simulink model "pendulum_on_cart"  (R2022a)
settings: Solver=VariableStepAuto  StartTime=0.0  StopTime=20  RelTol=1e-3
settings Model: Creator=Home  LastModifiedBy=Home

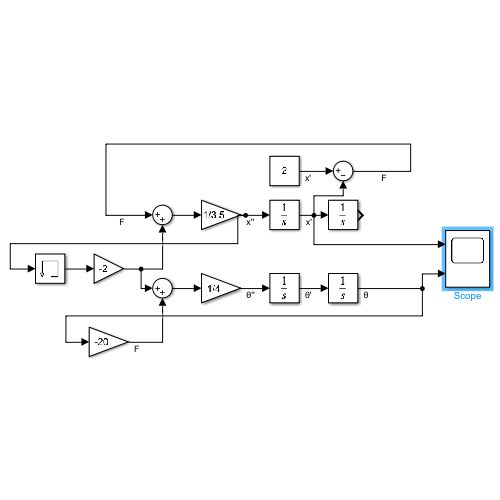
[thumbnail: Simulink's stored preview of the top-level diagram]
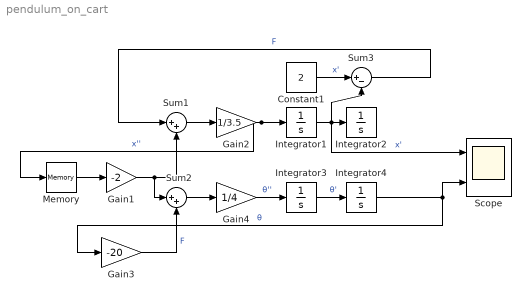
== system pendulum_on_cart ==
  Constant1 : Constant  Value=2
  Gain1 : Gain  Gain=-2
  Gain2 : Gain  Gain=1/3.5
  Gain3 : Gain  Gain=-20
  Gain4 : Gain  Gain=1/4
  Integrator{1..4} (4 alike) : Integrator
  Memory : Memory
  Scope : Scope  NumInputPorts=2
  Sum1 : Sum  Inputs=|++
  Sum2 : Sum  Inputs=|++
  Sum3 : Sum  Inputs=|+-
  wires:
  Sum1/1 -> Gain2/1
  Gain2/1 -> Memory/1, Integrator1/1  "x''"
  Integrator1/1 -> Scope/1, Sum3/2, Integrator2/1  "x'"
  Gain1/1 -> Sum2/1, Sum1/2
  Gain3/1 -> Sum2/2  "F"
  Sum2/1 -> Gain4/1
  Gain4/1 -> Integrator3/1  "θ''"
  Integrator3/1 -> Integrator4/1  "θ'"
  Integrator4/1 -> Scope/2, Gain3/1  "θ"
  Constant1/1 -> Sum3/1  "x'"
  Sum3/1 -> Sum1/1  "F"
  Memory/1 -> Gain1/1
